simulink model "phasofeederk2"  (Simulink 8.4)
settings: Solver=ode4  StartTime=0.0  StopTime=8  FixedStep=Ts  RelTol=1e-3
PreLoadFcn:
  | Ts=0.01;
PostLoadFcn:
  | Ts=0.01;
InitFcn:
  | Ts=0.01;
StartFcn:
  | Ts=0.01;
libraries: opal_lib x1, rtlab_phasor x1, rtlab x1
settings Model: Creator=ZhiqiZhao  LastModifiedBy=mchamana
settings DebuggingCC: FcnCallInpInsideContextMsg=EnableAllAsWarning

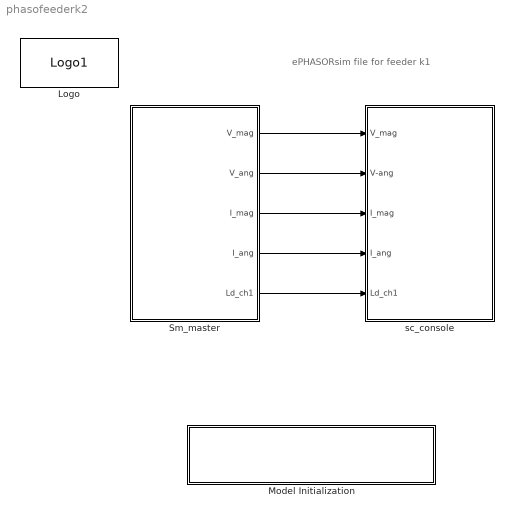
== system phasofeederk2 ==
  note: ePHASORsim file for
      | feeder k1
  Logo : opal_lib/Logo1  vide=[]
  Model Initialization : Subsystem  mask(Model Functions){InitFcnX=Ts=0.01;, prel=on, posl=on, inif=on, strf=on}
      mask prompts: InitFcnX "Initialisation"; prel "Preload Function"; posl "PostLoad Function"; inif "InitFcn"; strf "StartFcn"
      mask init:
      | currentBlock = gcb;
      | root = bdroot(currentBlock);
      | 
      | if ~strcmp(get_param(root,'BlockDiagramType'),'library')
      |     if prel==1
      |         set_param(root, 'PreLoadFcn', InitFcnX);
      |     else
      |         set_param(root, 'PreLoadFcn', '');
      |     end
      |     if inif==1
      |         set_param(root, 'InitFcn', InitFcnX);
      |     else
      |         set_param(root, 'InitFcn', '');
      |     end
      |     if strf==1
      |         set_param(root, 'StartFcn', InitFcnX);
      |     else
      |         set_param(root, 'StartFcn', '');
      |     end
      |     if posl==1
      |         set_param(root, 'PostLoadFcn', InitFcnX);
      |     else
      |         set_param(root, 'PostLoadFcn', '');
      |     end
      | end
      | 
      | pos = get_param(currentBlock, 'Position');
      | width = pos(3) - pos(1); height = pos(4) - pos(2);
      | txt = [ upper(root) '\n' '- InitFcn. . . . . '  get_param(root, 'InitFcn') ];
      settings: CopyFcn=set_param(gcb,'LinkStatus','none')
      mask Display: text(5, height*0.5, txt, 'horizontalAlignment', 'left', 'verticalAlignment', 'middle') ;
  Sm_master : Subsystem
  sc_console : Subsystem
  wires:
  Sm_master/1(V_mag) -> sc_console/1(V_mag)
  Sm_master/2(V_ang) -> sc_console/2(V-ang)
  Sm_master/5(Ld_ch1) -> sc_console/5(Ld_ch1)
  Sm_master/3(I_mag) -> sc_console/3(I_mag)
  Sm_master/4(I_ang) -> sc_console/4(I_ang)

== system phasofeederk2/Model Initialization ==

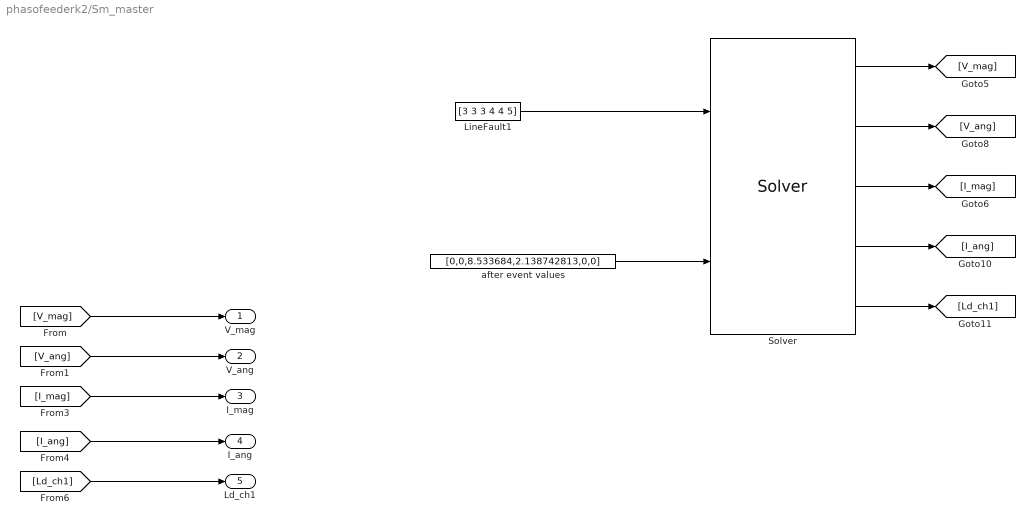
== system phasofeederk2/Sm_master ==
  LineFault1 : Constant  Value=[3 3 3 4 4 5]
  Solver : rtlab_phasor/Solver  extension=Excel  xls='phasor08_k1_mano1.xlsx'  raw='4992b.raw'  dyr='4992b.dyr'  cyme='typical.sxst'  cyme_pf=''  builtin_psse=on  lazy_netlist=on  capidir='CAPI'  fmudir='FMU'  capiprefix=capicomp_  fmuprefix=fmucomp_  logging=off  sim_mode=Dynamic simulation only (without power-flow)  pf_max_it=100  pf_tol_v=0.00000001  pf_export=on  np=1  exporty=off  dt=Ts  optim_threads=on  script_activate_postinit=off  script_postinit_name=''  script_activate_console=off
  after event values : Constant  Value=[0,0,8.533684,2.138742813,0,0]
  V_mag : Outport
  V_ang : Outport  Port=2
  I_mag : Outport  Port=3
  I_ang : Outport  Port=4
  Ld_ch1 : Outport  Port=5
  wires:
  LineFault1/1 -> Solver/1
  Solver/1 -> [V_mag]
  Solver/2 -> [V_ang]
  Solver/3 -> [I_mag]
  Solver/4 -> [I_ang]
  Solver/5 -> [Ld_ch1]
  after event values/1 -> Solver/2
  [V_mag] -> V_mag/1
  [V_ang] -> V_ang/1
  [I_ang] -> I_ang/1
  [I_mag] -> I_mag/1
  [Ld_ch1] -> Ld_ch1/1

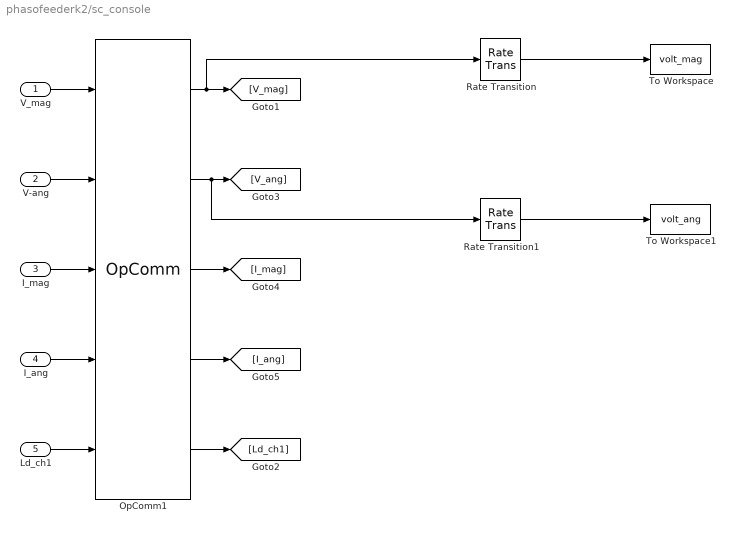
== system phasofeederk2/sc_console ==
  V_mag : Inport
  V-ang : Inport  Port=2
  I_mag : Inport  Port=3
  I_ang : Inport  Port=4
  Ld_ch1 : Inport  Port=5
  OpComm1 : rtlab/OpComm  nbport=5  groupe_acq=1  subsys_rate=0  st=0  Synchronization=on  Interpolation=on  Threshold=1.0  Missed_Data=off  Sim_Time=off  Samples=off  dynSigOut=off  from_console=0  warning_done=off  writeOpCommFile=off  Offset=off
  Rate Transition : RateTransition
  Rate Transition1 : RateTransition
  To Workspace : ToWorkspace  VariableName=volt_mag  SampleTime=1
  To Workspace1 : ToWorkspace  VariableName=volt_ang  SampleTime=1
  wires:
  V-ang/1 -> OpComm1/2
  V_mag/1 -> OpComm1/1
  OpComm1/1 -> Rate Transition/1, [V_mag]
  OpComm1/5 -> [Ld_ch1]
  Ld_ch1/1 -> OpComm1/5
  I_mag/1 -> OpComm1/3
  I_ang/1 -> OpComm1/4
  OpComm1/4 -> [I_ang]
  OpComm1/3 -> [I_mag]
  Rate Transition/1 -> To Workspace/1
  Rate Transition1/1 -> To Workspace1/1
  OpComm1/2 -> Rate Transition1/1, [V_ang]
